simulink library "sparten3e500kpq208c4_lib"  (R2013b)
settings: Solver=ode45  StartTime=0.0  StopTime=10.0  RelTol=1e-3
libraries: xbsIndex_r4 x5
settings Model: Creator=laca  LastModifiedBy=laca

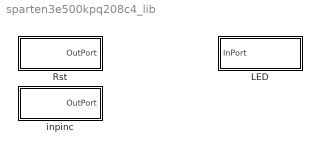
== system sparten3e500kpq208c4_lib ==
  LED : Subsystem  mask(Non-Memory-Mapped Output Port){show_out=off}
      mask prompts: show_out "Provide Output Double"
      mask help:
      | Port Name: "LED"
      | Port Type: 4-bit Vector
      mask init:
      | [bg,fg] = xlcmap('IO',0);
      | iPos = get_param(gcb,'Position');
      | iWidth=iPos(3)-iPos(1);
      | iHeight=iPos(4)-iPos(2);
      | [logoX, logoY] = xlogo(iPos);
      | if (show_out)
      |     old = find_system(gcb, 'LookUnderMasks', 'all', 'Name', 'Terminator');
      |     if (length(old) > 0)
      |         replace_block(gcb, 'Name', 'Terminator', 'OutPort', 'noprompt');
      |         set_param([gcb '/Terminator'], 'Name', 'OutPort');
      |     end
      |     portdir = 'output';
      |     portstr = 'dbl';
      | else
      |     old = find_system(gcb, 'LookUnderMasks', 'all', 'name', 'OutPort');
      |     if (length(old) > 0)
      |         replace_block(gcb, 'Name', 'OutPort', 'Terminator', 'noprompt');
      |         set_param([gcb '/OutPort'], 'Name', 'Terminator');
      |     end
      |     portdir = 'input';
      |     portstr = '';
      | end
      settings: CopyFcn=set_param(gcb,'LinkStatus','inactive');
      mask Display:
      | patch([0 iWidth iWidth 0],[0 0 iHeight iHeight] , bg);
      | patch(logoX,logoY, fg);
      | plot([0 0 iWidth iWidth 0], [0 iHeight iHeight 0 0]);
      | port_label(portdir,1,portstr);
      | port_label('input',1,'LED');
      | text(iWidth-10,5,'nmm');
  Rst : Subsystem  mask(Non-Memory-Mapped Input Port){signed=off, bpt=0, show_in=off, c=0}
      mask prompts: signed "Signed  (2's comp)"; bpt "Binary Point"; show_in "Provide Input Double"; c "Constant for Simulation"
      mask help:
      | Port Name: "Rst"
      | Port Type: Boolean
      mask init:
      | [bg,fg] = xlcmap('IO',0);
      | iPos = get_param(gcb,'Position');
      | iWidth=iPos(3)-iPos(1);
      | iHeight=iPos(4)-iPos(2);
      | [logoX, logoY] = xlogo(iPos);
      | if (show_in)
      |     old = find_system(gcb, 'LookUnderMasks', 'all', 'Name', 'Constant');
      |     if (length(old) > 0)
      |         replace_block(gcb, 'Name', 'Constant', 'InPort', 'noprompt');
      |         set_param([gcb '/Constant'], 'Name', 'InPort');
      |     end
      |     portdir = 'input';
      |     portstr = 'dbl';
      | else
      |     old = find_system(gcb, 'LookUnderMasks', 'all', 'Name', 'InPort');
      |     if (length(old) > 0)
      |         replace_block(gcb, 'Name', 'InPort', 'Constant', 'noprompt');
      |         set_param([gcb '/InPort'], 'Name', 'Constant');
      |         set_param([gcb '/Constant'], 'Value', 'c');
      |     end
      |     portdir = 'output';
      |     portstr = '';
      | end
      settings: CopyFcn=set_param(gcb,'LinkStatus','inactive');
      mask Callback show_in:
      | mask_vis = get_param(gcb, 'MaskVisibilities');
      | if (strcmp(get_param(gcb, 'show_in'),'on'))
      |     mask_vis(4) = {'off'};
      | else
      |     mask_vis(4) = {'on'};
      | end
      | set_param(gcb, 'MaskVisibilities', mask_vis);
      mask Display:
      | patch([0 iWidth iWidth 0],[0 0 iHeight iHeight] , bg);
      | patch(logoX,logoY, fg);
      | plot([0 0 iWidth iWidth 0], [0 iHeight iHeight 0 0]);
      | port_label(portdir,1,portstr);
      | port_label('output',1,'Rst');
      | text(2,5,'nmm');
  inpinc : Subsystem  mask(Non-Memory-Mapped Input Port){signed=off, bpt=0, show_in=off, c=0}
      mask prompts: signed "Signed  (2's comp)"; bpt "Binary Point"; show_in "Provide Input Double"; c "Constant for Simulation"
      mask help:
      | Port Name: "inpinc"
      | Port Type: 2-bit Vector
      mask init:
      | [bg,fg] = xlcmap('IO',0);
      | iPos = get_param(gcb,'Position');
      | iWidth=iPos(3)-iPos(1);
      | iHeight=iPos(4)-iPos(2);
      | [logoX, logoY] = xlogo(iPos);
      | if (signed)
      |     set_param([gcb '/inpinc'],'arith_type','Signed  (2''s comp)');
      | else
      |     set_param([gcb '/inpinc'],'arith_type','Unsigned');
      | end
      | if (show_in)
      |     old = find_system(gcb, 'LookUnderMasks', 'all', 'Name', 'Constant');
      |     if (length(old) > 0)
      |         replace_block(gcb, 'Name', 'Constant', 'InPort', 'noprompt');
      |         set_param([gcb '/Constant'], 'Name', 'InPort');
      |     end
      |     portdir = 'input';
      |     portstr = 'dbl';
      | else
      |     old = find_system(gcb, 'LookUnderMasks', 'all', 'Name', 'InPort');
      |     if (length(old) > 0)
      |         replace_block(gcb, 'Name', 'InPort', 'Constant', 'noprompt');
      |         set_param([gcb '/InPort'], 'Name', 'Constant');
      |         set_param([gcb '/Constant'], 'Value', 'c');
      |     end
      |     portdir = 'output';
      |     portstr = '';
      | end
      settings: CopyFcn=set_param(gcb,'LinkStatus','inactive');
      mask Callback show_in:
      | mask_vis = get_param(gcb, 'MaskVisibilities');
      | if (strcmp(get_param(gcb, 'show_in'),'on'))
      |     mask_vis(4) = {'off'};
      | else
      |     mask_vis(4) = {'on'};
      | end
      | set_param(gcb, 'MaskVisibilities', mask_vis);
      mask Display:
      | patch([0 iWidth iWidth 0],[0 0 iHeight iHeight] , bg);
      | patch(logoX,logoY, fg);
      | plot([0 0 iWidth iWidth 0], [0 iHeight iHeight 0 0]);
      | port_label(portdir,1,portstr);
      | port_label('output',1,'inpinc');
      | text(2,5,'nmm');

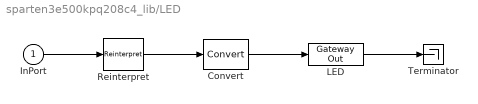
== system sparten3e500kpq208c4_lib/LED ==
  InPort : Inport
  Convert : xbsIndex_r4/Convert  gui_display_data_type=Fixed-point  arith_type=Unsigned  n_bits=4  bin_pt=0  float_type=Single  exp_bits=8  fraction_bits=24  quantization=Truncate  overflow=Wrap  en=off  latency=0  dbl_ovrd=off  pipeline=off  block_type=convert
  LED : xbsIndex_r4/Gateway Out  inherit_from_input=off  hdl_port=on  timing_constraint=None  locs_specified=on  LOCs={'P89','P83','P78','P68'}  UseAsDAC=off  DACChannel='1'  block_type=gatewayout
      settings: sginterface={'Xilinx'=>{'jtaghwcosim'=>{'non_memory_mapped_port'=>'LED'}}}
  Reinterpret : xbsIndex_r4/Reinterpret  force_arith_type=off  arith_type=Unsigned  force_bin_pt=off  bin_pt=0  block_type=reinterpret
  Terminator : Terminator
  wires:
  InPort/1 -> Reinterpret/1
  Reinterpret/1 -> Convert/1
  Convert/1 -> LED/1
  LED/1 -> Terminator/1

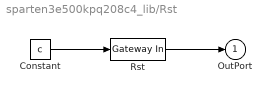
== system sparten3e500kpq208c4_lib/Rst ==
  Constant : Constant  Value=c
  Rst : xbsIndex_r4/Gateway In  gui_display_data_type=Fixed-point  arith_type=Boolean  n_bits=16  bin_pt=14  preci_type=Single  exp_width=8  frac_width=24  quantization="Round  (unbiased: +/- Inf)"  overflow=Saturate  period=1  dbl_ovrd=off  timing_constraint=None  locs_specified=on  LOCs={'P101'}  UseAsADC=off  ADCChannel='1'  inherit_from_input=off  hdl_port=on  block_type=gatewayin
      settings: sginterface={'Xilinx'=>{'jtaghwcosim'=>{'non_memory_mapped_port'=>'Rst'}}}
  OutPort : Outport
  wires:
  Constant/1 -> Rst/1
  Rst/1 -> OutPort/1

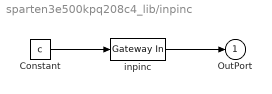
== system sparten3e500kpq208c4_lib/inpinc ==
  Constant : Constant  Value=c
  inpinc : xbsIndex_r4/Gateway In  gui_display_data_type=Fixed-point  arith_type=Unsigned  n_bits=2  bin_pt=max(0,min(bpt,2))  preci_type=Single  exp_width=8  frac_width=24  quantization="Round  (unbiased: +/- Inf)"  overflow=Saturate  period=1  dbl_ovrd=off  timing_constraint=None  locs_specified=on  LOCs={'P116','P119'}  UseAsADC=off  ADCChannel='1'  inherit_from_input=off  hdl_port=on  block_type=gatewayin
      settings: sginterface={'Xilinx'=>{'jtaghwcosim'=>{'non_memory_mapped_port'=>'inpinc'}}}
  OutPort : Outport
  wires:
  Constant/1 -> inpinc/1
  inpinc/1 -> OutPort/1
